simulink model "backup"  (R2017a)
settings: Solver=FixedStepDiscrete  StartTime=0.0  StopTime=inf  RelTol=1e-3  EnableMultiTasking=on
undefined symbols (not defined in the file or in its folder): fspecial, gray, Rec, SDTV, strel
libraries: simulink x11, visiontransforms x4, visionmorphops x3, visiontextngfix x3, visiongeotforms x2, visionsources x2, visionconversions x1, visionutilities x1, dspvision x1, visionstatistics x1, visionfilter x1
settings Model: FPTRunName=Active  Creator=The MathWorks, Inc.  LastModifiedBy=Pection
settings DataIOCC: LimitDataPoints=on  SaveFormat=StructureWithTime  SaveOutput=off  SignalLogging=off  SaveTime=off
settings OptimizationCC: ExpressionDepthLimit=2147483647  InitFltsAndDblsToZero=on  EfficientMapNaN2IntZero=off  LifeSpan=inf
settings DebuggingCC: UnderspecifiedInitializationDetection=Classic  MergeDetectMultiDrivingBlocksExec=none  SolverPrmCheckMsg=warning  ParameterPrecisionLossMsg=none  FcnCallInpInsideContextMsg=warning  StateNameClashWarn=warning  SFUnexpectedBacktrackingDiag=warning  SFNoUnconditionalDefaultTransitionDiag=warning  SFExecutionAtInitializationDiag=none
settings HardwareCC: ProdBitPerPointer=32  ProdBitPerSizeT=32  ProdBitPerPtrDiffT=32  ProdLargestAtomicFloat=None  ProdIntDivRoundTo=Undefined  ProdEndianess=Unspecified  ProdWordSize=32  ProdHWDeviceType=32-bit Generic  TargetBitPerPointer=64  TargetBitPerSizeT=64  TargetBitPerPtrDiffT=64  TargetLongLongMode=on  TargetIntDivRoundTo=Zero  TargetEndianess=LittleEndian  TargetWordSize=64  TargetHWDeviceType=Generic->MATLAB Host Computer  ProdEqTarget=off
settings ModelReferenceCC: PropagateSignalLabelsOutOfModel=off
settings SFSimCC: SimParseCustomCode=off
settings GRTTargetCC: TargetLangStandard=C89/C90 (ANSI)  GeneratePreprocessorConditionals=Disable all  CombineOutputUpdateFcns=off  GRTInterface=on
settings ConfigComp: CovMetricSettings=dw  CovHtmlReporting=on  CovSaveCumulativeToWorkspaceVar=on  CovSaveSingleToWorkspaceVar=on  CovExternalEMLEnable=off  CovSFcnEnable=off

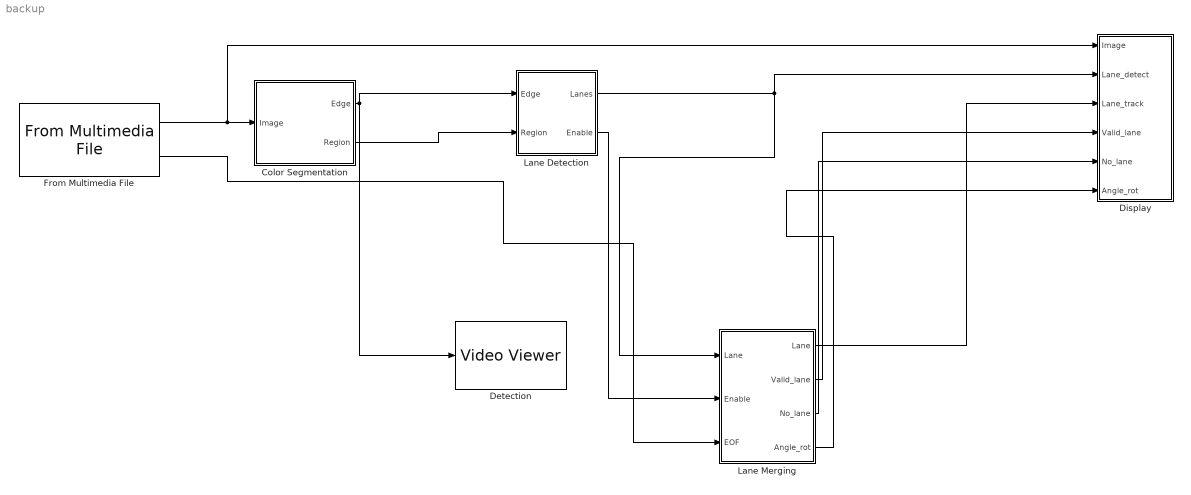
== system backup ==
  Color Segmentation : Subsystem
  Detection : VideoViewer  colormapValue=gray(256)  FigPos=[1 1038 1920 938]  trueSizedOnce=on
  Display : Subsystem
  From Multimedia File : dspvision/From Multimedia File  inputFilename=C:\Users\Pection\Desktop\vipunmarkedroad.avi  loop=on  numPlays=inf  outputStreams=Video only  videoDataType=single  audioDataType=int16  inheritSampleTime=off  userDefinedSampleTime=1/30  noAudioOutput=off  isIntensityVideo=off  fourcc=RGB  colorVideoFormat=One multidimensional signal  outputEOF=on  dataOrg=Column-major  audioFrameSize=1024  computeAudioFrameSize=off  outSamplingMode=Frame based
      settings: SourceProductBaseCode=VP
  Lane Detection : Subsystem
  Lane Merging : Subsystem
  wires:
  From Multimedia File/1 -> Display/1(Image), Color Segmentation/1(Image)
  Color Segmentation/2(Region) -> Lane Detection/2(Region)
  From Multimedia File/2 -> Lane Merging/3(EOF)
  Lane Detection/1(Lanes) -> Display/2(Lane_detect), Lane Merging/1(Lane)
  Lane Detection/2(Enable) -> Lane Merging/2(Enable)
  Lane Merging/1("Lane ") -> Display/3(Lane_track)
  Lane Merging/2(Valid_lane) -> Display/4(Valid_lane)
  Lane Merging/3(No_lane) -> Display/5(No_lane)
  Lane Merging/4(Angle_rot) -> Display/6(Angle_rot)
  Color Segmentation/1(Edge) -> Detection/1, Lane Detection/1(Edge)

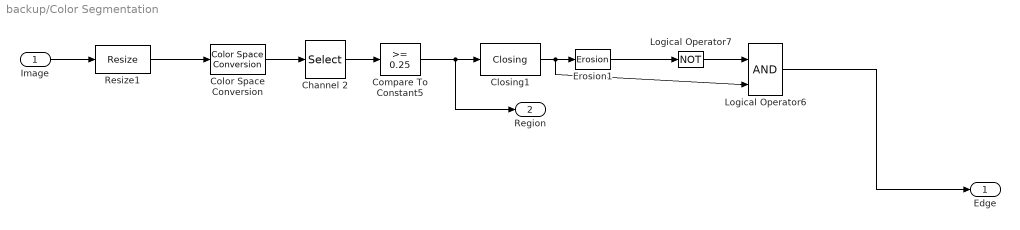
== system backup/Color Segmentation ==
  Image : Inport
  Channel 2 : Selector  NumberOfDimensions=3  InputPortWidth=3  IndexOptions=Select all,Select all,Index vector (dialog)  Indices=[1 3],1,[2]  OutputSizes=1,1,1
  Closing1 : visionmorphops/Closing  nhoodsrc=Specify via dialog  strel=strel('disk', 2)
      settings: SourceProductName=Computer Vision System Toolbox  SourceProductBaseCode=VP
  Color Space Conversion : visionconversions/Color Space  Conversion  conversion=Obsolete  conversionActive=R'G'B' to HSV  wp_str=D65  rec=Rec. 601 (SDTV)  sys=1125/60/2:1  imagePorts=One multidimensional signal
      settings: SourceProductName=Computer Vision System Toolbox
  Compare To Constant5 : simulink/Logic and Bit Operations/Compare To Constant  relop=>=  const=0.25  OutDataTypeStr=boolean  ZeroCross=off
  Erosion1 : visionmorphops/Erosion  nhoodsrc=Specify via dialog  strel=ones(3)
      settings: SourceProductName=Computer Vision System Toolbox  SourceProductBaseCode=VP
  Logical Operator6 : Logic  IconShape=distinctive  AllPortsSameDT=off  OutDataTypeStr=boolean
  Logical Operator7 : Logic  Operator=NOT  IconShape=distinctive  AllPortsSameDT=off  OutDataTypeStr=boolean
  Resize1 : visiongeotforms/Resize  specify=Output size as a percentage of input size  rfactor=50  outCols=25  outRows=25  outRowsCols=[120 160]  interp_method=Nearest neighbor  antialias=off  useROI=off  roiFlag=off  prodOutputMode=Binary point scaling  prodOutputWordLength=32  prodOutputFracLength=10  roundingMode=Nearest  overflowMode=on
      settings: AttributesFormatString=Downsample the\ninput image to\nreduce computation.  SourceProductName=Computer Vision System Toolbox  SourceProductBaseCode=VP
  Edge : Outport
  Region : Outport  Port=2
  wires:
  Color Space Conversion/1 -> Channel 2/1
  Channel 2/1 -> Compare To Constant5/1
  Closing1/1 -> Erosion1/1, Logical Operator6/2
  Logical Operator7/1 -> Logical Operator6/1
  Erosion1/1 -> Logical Operator7/1
  Compare To Constant5/1 -> Region/1, Closing1/1
  Image/1 -> Resize1/1
  Logical Operator6/1 -> Edge/1
  Resize1/1 -> Color Space Conversion/1

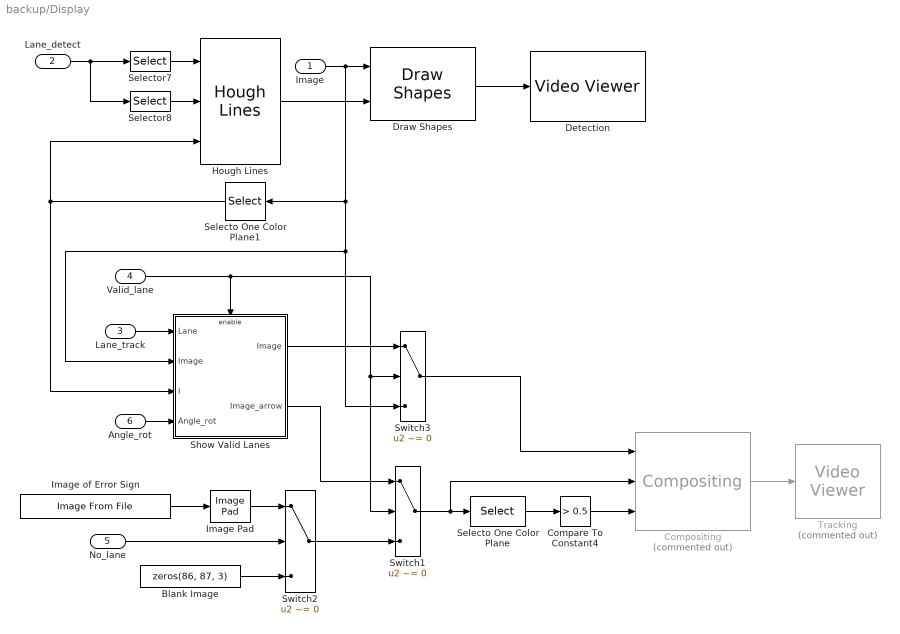
== system backup/Display ==
  Image : Inport
  Lane_detect : Inport  Port=2
  Lane_track : Inport  Port=3
  Valid_lane : Inport  Port=4
  No_lane : Inport  Port=5
  Angle_rot : Inport  Port=6
  Blank Image : Constant  Value=zeros(86, 87, 3)  OutDataTypeStr=Inherit: Inherit via back propagation
  Compare To Constant4 : simulink/Logic and Bit Operations/Compare To Constant  relop=>  const=0.5  OutDataTypeStr=uint8  ZeroCross=off
  Compositing : visiontextngfix/Compositing  Commented=on  operation=Binary mask  bFacSrc=Specify via dialog  mFacSrc=Input port  bFactor=0.75  mFactor=1  source=Specify via dialog  coordinates=[110 140]  prodOutputMode=Binary point scaling  prodOutputWordLength=32  prodOutputFracLength=10  roundingMode=Floor  overflowMode=off
      settings: SourceProductName=Computer Vision System Toolbox  SourceProductBaseCode=VP
  Detection : VideoViewer  colormapValue=gray(256)  FigPos=[169 782 575 518]  trueSizedOnce=on
  Draw Shapes : visiontextngfix/Draw Shapes  shape=Lines  fill=off  lineWidth=1  fillClrSource=Specify via dialog  display=User-specified value  intensity=200  color=[1 1 0; 1 0 1]  opacity=0.6  viewport=Entire image  antialiasing=off  inType=Obsolete  imagePorts=One multidimensional signal  prodOutputMode=Binary point scaling  prodOutputWordLength=32  prodOutputFracLength=14  memoryMode=Specify word length  memoryWordLength=16  memoryFracLength=15  roundingMode=Floor  overflowMode=off
      settings: SourceProductName=Computer Vision System Toolbox
  Hough Lines : visiontransforms/Hough Lines  sineCompMethod=Trigonometric function  thetaRes=pi/180  firstCoeffMode=Specify word length  firstCoeffWordLength=16  firstCoeffFracLength=15  prodOutputMode=Binary point scaling  prodOutputWordLength=32  prodOutputFracLength=16  roundingMode=Nearest  overflowMode=on
      settings: SourceProductName=Computer Vision System Toolbox  SourceProductBaseCode=VP
  Image Pad : visionutilities/Image Pad  method=Constant  valSrc=Specify via dialog  value=0  spec=Output size  rowDirection=Right  outRowsMode=User-specified  rowSize=86  outColSize=87  colDirection=Bottom  outColsMode=User-specified  colSize=87  outRowSize=86  trunc_flag=None
      settings: SourceProductName=Computer Vision System Toolbox  SourceProductBaseCode=VP
  Image of Error Sign : visionsources/Image From File  Tag=vipblks_nd  FileName=viperrorsign.png  imagePorts=One multidimensional signal  Ts=inf  ImageDataType=single  Signed=on  WordLength=16  sdImageDataType=uint(8)  FractionLengthMode=User-defined  FractionLength=15  OutPortLabels=R|G|B
      settings: SourceProductName=Computer Vision System Toolbox
  Selecto One Color Plane : Selector  NumberOfDimensions=3  IndexMode=Zero-based  InputPortWidth=3  IndexOptions=Select all,Select all,Index vector (dialog)  Indices=[1 3],1,0  OutputSizes=1,1,1
  Selecto One Color Plane1 : Selector  NumberOfDimensions=3  IndexMode=Zero-based  InputPortWidth=3  IndexOptions=Select all,Select all,Index vector (dialog)  Indices=[1 3],1,0  OutputSizes=1,1,1
  Selector7 : Selector  NumberOfDimensions=2  IndexMode=Zero-based  InputPortWidth=2  IndexOptions=Index vector (dialog),Select all  Indices=1,0  OutputSizes=1,1
  Selector8 : Selector  NumberOfDimensions=2  IndexMode=Zero-based  InputPortWidth=2  IndexOptions=Index vector (dialog),Select all  Indices=0,0  OutputSizes=1,1
  Show Valid Lanes : Subsystem
  Switch1 : Switch  Criteria=u2 ~= 0
  Switch2 : Switch  Criteria=u2 ~= 0
  Switch3 : Switch  Criteria=u2 ~= 0
  Tracking : VideoViewer  Commented=on  colormapValue=gray(256)  FigPos=[852 826 725 493]  trueSizedOnce=on
  wires:
  Hough Lines/1 -> Draw Shapes/2
  Image/1 -> Draw Shapes/1, Switch3/3, Show Valid Lanes/2(Image), Selecto One Color Plane1/1
  Draw Shapes/1 -> Detection/1
  Selector7/1 -> Hough Lines/1
  Selector8/1 -> Hough Lines/2
  Selecto One Color Plane/1 -> Compare To Constant4/1
  Compare To Constant4/1 -> Compositing/3
  Blank Image/1 -> Switch2/3
  Image of Error Sign/1 -> Image Pad/1
  Switch2/1 -> Switch1/3
  Compositing/1 -> Tracking/1
  Image Pad/1 -> Switch2/1
  Lane_detect/1 -> Selector7/1, Selector8/1
  Switch3/1 -> Compositing/1
  Show Valid Lanes/1("Image ") -> Switch3/1
  Show Valid Lanes/2(Image_arrow) -> Switch1/1
  No_lane/1 -> Switch2/2
  Switch1/1 -> Selecto One Color Plane/1, Compositing/2
  Lane_track/1 -> Show Valid Lanes/1(Lane)
  Angle_rot/1 -> Show Valid Lanes/4(Angle_rot)
  Valid_lane/1 -> Show Valid Lanes/Enable, Switch3/2, Switch1/2
  Selecto One Color Plane1/1 -> Hough Lines/3, Show Valid Lanes/3(I)

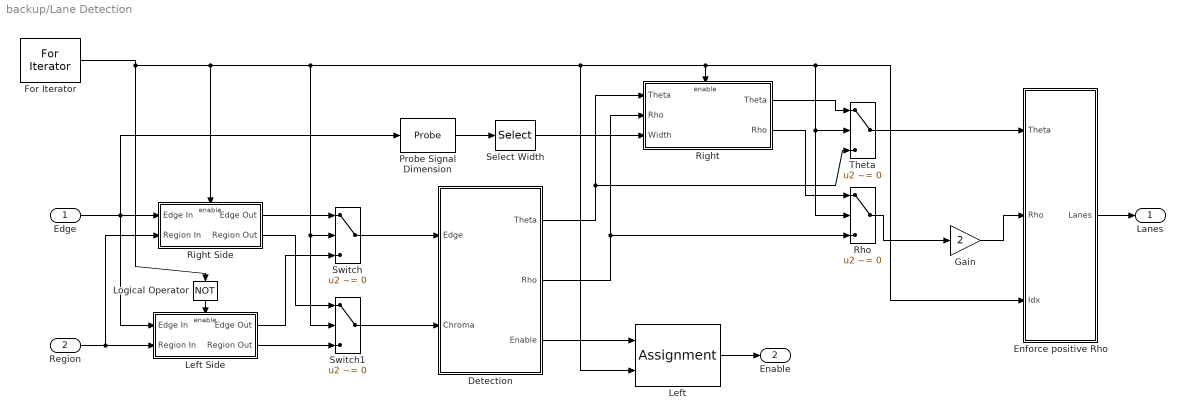
== system backup/Lane Detection ==
  Edge : Inport
  Region : Inport  Port=2
  Detection : Subsystem
  Enforce positive Rho : Subsystem
  For Iterator : ForIterator  IterationLimit=2  IndexMode=Zero-based  IterationVariableDataType=int8
  Gain : Gain  Gain=2
  Left : Assignment  NumberOfDimensions=2  IndexMode=Zero-based  OutputInitialize=Specify size for each dimension in table  IndexOptions=Assign all,Index vector (port)  Indices=1,1  OutputSizes=1,2
  Left Side : Subsystem  TreatAsAtomicUnit=on
  Logical Operator : Logic  Operator=NOT  IconShape=distinctive  AllPortsSameDT=off  OutDataTypeStr=boolean
  Probe Signal Dimension : Probe  ProbeWidth=off  ProbeSampleTime=off  ProbeComplexSignal=off  ProbeSignalDimensions=on  ProbeDimensionsDataType=single
  Rho : Switch  Criteria=u2 ~= 0
  Right : Subsystem  TreatAsAtomicUnit=on
  Right Side : Subsystem  TreatAsAtomicUnit=on
  Select Width : Selector  IndexMode=Zero-based  InputPortWidth=2  IndexOptions=Index vector (dialog)  Indices=1  OutputSizes=1
  Switch : Switch  Criteria=u2 ~= 0
  Switch1 : Switch  Criteria=u2 ~= 0
  Theta : Switch  Criteria=u2 ~= 0
  Lanes : Outport
  Enable : Outport  Port=2
  wires:
  Logical Operator/1 -> Left Side/Enable
  For Iterator/1 -> Logical Operator/1, Right Side/Enable, Switch/2, Switch1/2, Right/Enable, Enforce positive Rho/3(Idx), Theta/2, Rho/2, Left/2
  Edge/1 -> Right Side/1(Edge In), Left Side/1(Edge In), Probe Signal Dimension/1
  Region/1 -> Left Side/2(Region In), Right Side/2(Region In)
  Switch/1 -> Detection/1(Edge)
  Right Side/1(Edge Out) -> Switch/1
  Left Side/1(Edge Out) -> Switch/3
  Switch1/1 -> Detection/2(Chroma)
  Right Side/2(Region Out) -> Switch1/1
  Left Side/2("Region Out ") -> Switch1/3
  Left/1 -> Enable/1
  Right/1("Theta ") -> Theta/1
  Right/2("Rho ") -> Rho/1
  Enforce positive Rho/1(Lanes) -> Lanes/1
  Detection/3(Enable) -> Left/1
  Theta/1 -> Enforce positive Rho/1(Theta)
  Rho/1 -> Gain/1
  Detection/1(Theta) -> Right/1(Theta), Theta/3
  Detection/2(Rho) -> Right/2(Rho), Rho/3
  Gain/1 -> Enforce positive Rho/2(Rho)
  Probe Signal Dimension/1 -> Select Width/1
  Select Width/1 -> Right/3(Width)

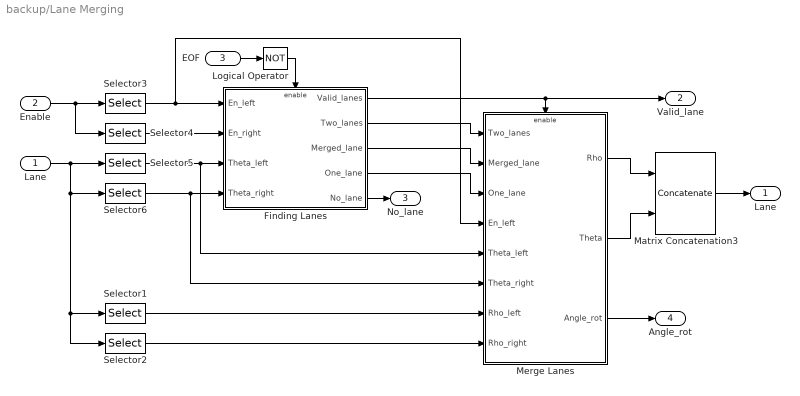
== system backup/Lane Merging ==
  Lane : Inport
  Enable : Inport  Port=2
  EOF : Inport  Port=3
  Finding Lanes : Subsystem  mask{appearTime=4}
      mask prompts: appearTime "Minimum number of frames a lane must be detected to become a valid lane:"
  Logical Operator : Logic  Operator=NOT  IconShape=distinctive  AllPortsSameDT=off  OutDataTypeStr=boolean
  Matrix Concatenation3 : Concatenate  Mode=Multidimensional array
  Merge Lanes : Subsystem
  Selector1 : Selector  NumberOfDimensions=2  IndexMode=Zero-based  InputPortWidth=2  IndexOptions=Index vector (dialog),Index vector (dialog)  Indices=0,0  OutputSizes=1,1
  Selector2 : Selector  NumberOfDimensions=2  IndexMode=Zero-based  InputPortWidth=2  IndexOptions=Index vector (dialog),Index vector (dialog)  Indices=0,1  OutputSizes=1,1
  Selector3 : Selector  IndexMode=Zero-based  InputPortWidth=2  IndexOptions=Index vector (dialog)  Indices=0  OutputSizes=1
  Selector4 : Selector  IndexMode=Zero-based  InputPortWidth=2  IndexOptions=Index vector (dialog)  Indices=1  OutputSizes=1
  Selector5 : Selector  NumberOfDimensions=2  IndexMode=Zero-based  InputPortWidth=2  IndexOptions=Index vector (dialog),Index vector (dialog)  Indices=1,0  OutputSizes=1,1
  Selector6 : Selector  NumberOfDimensions=2  IndexMode=Zero-based  InputPortWidth=2  IndexOptions=Index vector (dialog),Index vector (dialog)  Indices=1,1  OutputSizes=1,1
  "Lane " : Outport
  Valid_lane : Outport  Port=2
  No_lane : Outport  Port=3
  Angle_rot : Outport  Port=4
  wires:
  Enable/1 -> Selector3/1, Selector4/1
  Finding Lanes/2(Two_lanes) -> Merge Lanes/1(Two_lanes)
  Finding Lanes/3(Merged_lane) -> Merge Lanes/2(Merged_lane)
  Finding Lanes/4(One_lane) -> Merge Lanes/3(One_lane)
  EOF/1 -> Logical Operator/1
  Logical Operator/1 -> Finding Lanes/Enable
  Selector3/1 -> Finding Lanes/1(En_left), Merge Lanes/4(En_left)
  Selector4/1 -> Finding Lanes/2(En_right)
  Lane/1 -> Selector5/1, Selector6/1, Selector2/1, Selector1/1
  Selector5/1 -> Finding Lanes/3(Theta_left), Merge Lanes/5(Theta_left)
  Selector6/1 -> Finding Lanes/4(Theta_right), Merge Lanes/6(Theta_right)
  Finding Lanes/5(No_lane) -> No_lane/1
  Merge Lanes/3(Angle_rot) -> Angle_rot/1
  Finding Lanes/1(Valid_lanes) -> Merge Lanes/Enable, Valid_lane/1
  Merge Lanes/1("Rho ") -> Matrix Concatenation3/1
  Merge Lanes/2("Theta ") -> Matrix Concatenation3/2
  Matrix Concatenation3/1 -> "Lane "/1
  Selector1/1 -> Merge Lanes/7(Rho_left)
  Selector2/1 -> Merge Lanes/8(Rho_right)

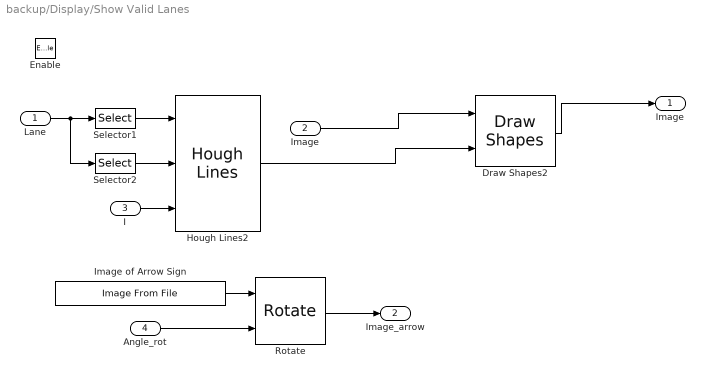
== system backup/Display/Show Valid Lanes ==
  Lane : Inport
  Image : Inport  Port=2
  I : Inport  Port=3
  Angle_rot : Inport  Port=4
  Enable : EnablePort  StatesWhenEnabling=reset  PropagateVarSize=During execution
  Draw Shapes2 : visiontextngfix/Draw Shapes  shape=Lines  fill=off  lineWidth=1  fillClrSource=Specify via dialog  display=User-specified value  intensity=200  color=[1 1 0; 1 0 1; 0 1 1]  opacity=0.6  viewport=Entire image  antialiasing=off  inType=Obsolete  imagePorts=One multidimensional signal  prodOutputMode=Binary point scaling  prodOutputWordLength=32  prodOutputFracLength=14  memoryMode=Specify word length  memoryWordLength=16  memoryFracLength=15  roundingMode=Floor  overflowMode=off
      settings: SourceProductName=Computer Vision System Toolbox
  Hough Lines2 : visiontransforms/Hough Lines  sineCompMethod=Trigonometric function  thetaRes=pi/180  firstCoeffMode=Specify word length  firstCoeffWordLength=16  firstCoeffFracLength=15  prodOutputMode=Binary point scaling  prodOutputWordLength=32  prodOutputFracLength=16  roundingMode=Nearest  overflowMode=on
      settings: SourceProductName=Computer Vision System Toolbox  SourceProductBaseCode=VP
  Image of Arrow Sign : visionsources/Image From File  Tag=vipblks_nd  FileName=viparrowsign.png  imagePorts=One multidimensional signal  Ts=inf  ImageDataType=single  Signed=on  WordLength=16  sdImageDataType=uint(8)  FractionLengthMode=User-defined  FractionLength=15  OutPortLabels=R|G|B
      settings: SourceProductName=Computer Vision System Toolbox
  Rotate : visiongeotforms/Rotate  outSizeR=Expanded to fit rotated input image  src_angle=Input port  unit_angle=Degrees  angle=pi/6  maxAngle=pi  dispImage=Center  method=Trigonometric function  fillVal=0  interpMethod=Bilinear  prodOutputMode=Binary point scaling  prodOutputWordLength=32  prodOutputFracLength=10  roundingMode=Nearest  overflowMode=on
      settings: SourceProductName=Computer Vision System Toolbox
  Selector1 : Selector  NumberOfDimensions=2  IndexMode=Zero-based  InputPortWidth=2  IndexOptions=Index vector (dialog),Select all  Indices=1,0  OutputSizes=1,1
  Selector2 : Selector  NumberOfDimensions=2  IndexMode=Zero-based  InputPortWidth=2  IndexOptions=Index vector (dialog),Select all  Indices=0,0  OutputSizes=1,1
  "Image " : Outport
  Image_arrow : Outport  Port=2
  wires:
  Hough Lines2/1 -> Draw Shapes2/2
  Image of Arrow Sign/1 -> Rotate/1
  Lane/1 -> Selector1/1, Selector2/1
  Selector1/1 -> Hough Lines2/1
  Selector2/1 -> Hough Lines2/2
  Angle_rot/1 -> Rotate/2
  Image/1 -> Draw Shapes2/1
  I/1 -> Hough Lines2/3
  Draw Shapes2/1 -> "Image "/1
  Rotate/1 -> Image_arrow/1

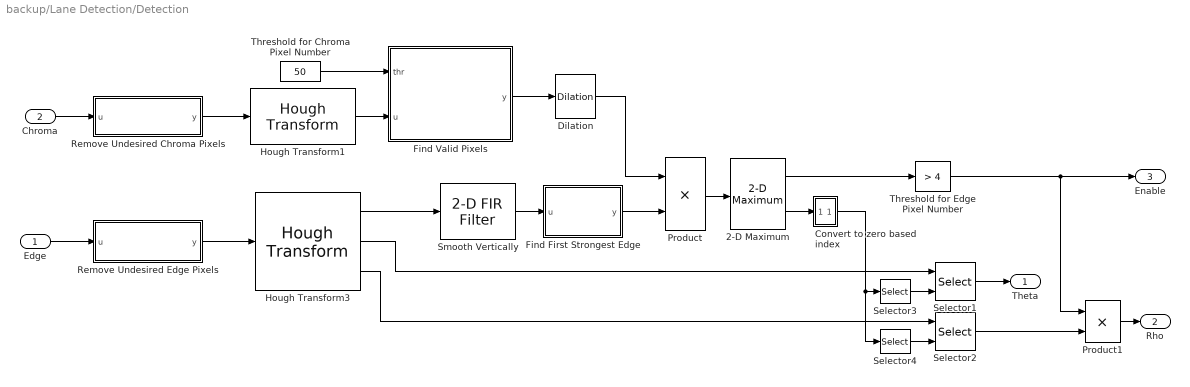
== system backup/Lane Detection/Detection ==
  Edge : Inport
  Chroma : Inport  Port=2
  2-D Maximum : visionstatistics/2-D Maximum  fcn=Value and Index  reset=None  indexBase=One  operateOver=Entire input  Dimension=1  colComp=on  operation=maximum  roiEnable=off  roiType=Rectangles  roiPortion=Entire ROI  roiOutput=Individual statistics for each ROI  roiFlag=off  accumDataTypeStr=Inherit: Same as product output  accumLastDataTypeStr=Inherit: Same as product output  roundingMode=Floor  overflowMode=off
      settings: SourceProductName=Computer Vision System Toolbox  SourceProductBaseCode=VP
  "Convert to zero based index " : Subsystem
  Dilation : visionmorphops/Dilation  nhoodsrc=Specify via dialog  strel=ones(3, 1)
      settings: SourceProductName=Computer Vision System Toolbox  SourceProductBaseCode=VP
  Find First Strongest Edge : MATLAB Function  TreatAsAtomicUnit=on
  Find Valid Pixels : MATLAB Function  TreatAsAtomicUnit=on
      settings: AttributesFormatString=Find valid pixels in each of the angles.
  Hough Transform1 : visiontransforms/Hough Transform  theta_res=pi/90  rho_res=2  out_theta_rho=off  outdtmode=single  firstCoeffMode=Binary point scaling  firstCoeffWordLength=16  firstCoeffFracLength=14  secondCoeffMode=Binary point scaling  secondCoeffWordLength=32  secondCoeffFracLength=16  outputMode=Binary point scaling  outputWordLength=16  outputFracLength=0  accumMode=Binary point scaling  accumWordLength=32  accumFracLength=20  prodOutputMode=Binary point scaling  prodOutputWordLength=32  prodOutputFracLength=20  memoryMode=Binary point scaling  memoryWordLength=32  memoryFracLength=16  roundingMode=Nearest  overflowMode=on
      settings: SourceProductName=Computer Vision System Toolbox  SourceProductBaseCode=VP
  Hough Transform3 : visiontransforms/Hough Transform  theta_res=pi/90  rho_res=2  out_theta_rho=on  outdtmode=single  firstCoeffMode=Binary point scaling  firstCoeffWordLength=16  firstCoeffFracLength=14  secondCoeffMode=Binary point scaling  secondCoeffWordLength=32  secondCoeffFracLength=16  outputMode=Binary point scaling  outputWordLength=16  outputFracLength=0  accumMode=Binary point scaling  accumWordLength=32  accumFracLength=20  prodOutputMode=Binary point scaling  prodOutputWordLength=32  prodOutputFracLength=20  memoryMode=Binary point scaling  memoryWordLength=32  memoryFracLength=16  roundingMode=Nearest  overflowMode=on
      settings: SourceProductName=Computer Vision System Toolbox  SourceProductBaseCode=VP
  Product : Product  RndMeth=Zero
  Product1 : Product  RndMeth=Zero
  Remove Undesired Chroma Pixels : MATLAB Function  TreatAsAtomicUnit=on
  Remove Undesired Edge Pixels : MATLAB Function  TreatAsAtomicUnit=on
  Selector1 : Selector  IndexMode=Zero-based  IndexOptions=Index vector (port)  Indices=[1 3]  OutputSizes=1
  Selector2 : Selector  IndexMode=Zero-based  IndexOptions=Index vector (port)  Indices=[1 3]  OutputSizes=1
  Selector3 : Selector  IndexMode=Zero-based  InputPortWidth=2  IndexOptions=Index vector (dialog)  Indices=1  OutputSizes=1
  Selector4 : Selector  IndexMode=Zero-based  InputPortWidth=2  IndexOptions=Index vector (dialog)  Indices=0  OutputSizes=1
  Smooth Vertically : visionfilter/2-D FIR Filter  separable=off  filtSrc=Specify via dialog  filterMtrx=fspecial('gaussian', [5, 1], 1.5)  verticalFilter=fspecial('gaussian', [7, 1] ,2)  horizontalFilter=1  outSize=Same as input port I  padType=Replicate  padSrc=Specify via dialog  padVal=0  method=Convolution  firstCoeffMode=Specify word length  firstCoeffWordLength=16  firstCoeffFracLength=17  firstCoeffSignedness=Signed  firstCoeffDataTypeStr=fixdt(1,16)  firstCoeffLastDataTypeStr=fixdt(1,16)  firstCoeffMin=[]  firstCoeffMax=[]  outputSignedness=Auto  outputMin=[]  outputMax=[]  accumDataTypeStr=Inherit: Same as product output  accumLastDataTypeStr=Inherit: Same as product output  prodOutputMode=Binary point scaling  prodOutputWordLength=32  prodOutputFracLength=10  prodOutputDataTypeStr=fixdt([],32,10)  prodOutputLastDataTypeStr=fixdt([],32,10)  roundingMode=Floor  overflowMode=off
      settings: SourceProductName=Computer Vision System Toolbox  SourceProductBaseCode=VP
  Threshold for Chroma Pixel Number : Constant  Value=50
  Threshold for Edge Pixel Number : simulink/Logic and Bit Operations/Compare To Constant  relop=>  const=4  OutDataTypeStr=uint8  ZeroCross=off
  Theta : Outport
  Rho : Outport  Port=2
  Enable : Outport  Port=3
  wires:
  Remove Undesired Edge Pixels/1(y) -> Hough Transform3/1
  Hough Transform3/1 -> Smooth Vertically/1
  Hough Transform3/2 -> Selector1/1
  Hough Transform3/3 -> Selector2/1
  Selector3/1 -> Selector1/2
  Selector4/1 -> Selector2/2
  Smooth Vertically/1 -> Find First Strongest Edge/1(u)
  2-D Maximum/1 -> Threshold for Edge Pixel Number/1
  Selector1/1 -> Theta/1
  Edge/1 -> Remove Undesired Edge Pixels/1(u)
  Chroma/1 -> Remove Undesired Chroma Pixels/1(u)
  Threshold for Edge Pixel Number/1 -> Product1/1, Enable/1
  Product1/1 -> Rho/1
  Selector2/1 -> Product1/2
  Find First Strongest Edge/1(y) -> Product/2
  Product/1 -> 2-D Maximum/1
  Hough Transform1/1 -> Find Valid Pixels/2(u)
  Find Valid Pixels/1(y) -> Dilation/1
  Remove Undesired Chroma Pixels/1(y) -> Hough Transform1/1
  Threshold for Chroma Pixel Number/1 -> Find Valid Pixels/1(thr)
  Dilation/1 -> Product/1
  2-D Maximum/2 -> "Convert to zero based index "/1(In1)
  "Convert to zero based index "/1(Out1) -> Selector3/1, Selector4/1

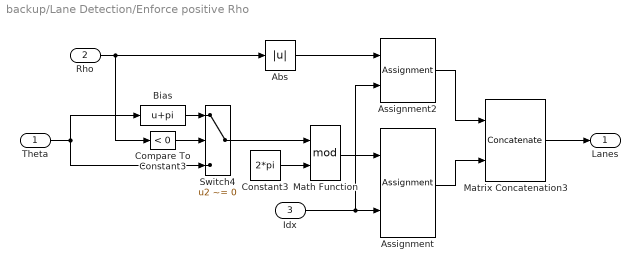
== system backup/Lane Detection/Enforce positive Rho ==
  Theta : Inport
  Rho : Inport  Port=2
  Idx : Inport  Port=3
  Abs : Abs
  Assignment : Assignment  NumberOfDimensions=2  IndexMode=Zero-based  OutputInitialize=Specify size for each dimension in table  IndexOptions=Assign all,Index vector (port)  Indices=1,1  OutputSizes=1,2
  Assignment2 : Assignment  NumberOfDimensions=2  IndexMode=Zero-based  OutputInitialize=Specify size for each dimension in table  IndexOptions=Assign all,Index vector (port)  Indices=1,1  OutputSizes=1,2
  Bias : Bias  Bias=pi
  Compare To Constant3 : simulink/Logic and Bit Operations/Compare To Constant  relop=<  const=0  OutDataTypeStr=uint8  ZeroCross=off
  Constant3 : Constant  Value=2*pi  OutDataTypeStr=Inherit: Inherit via back propagation
  Math Function : Math  Operator=mod  SaturateOnIntegerOverflow=on
  Matrix Concatenation3 : Concatenate  Mode=Multidimensional array
  Switch4 : Switch  Criteria=u2 ~= 0
  Lanes : Outport
  wires:
  Theta/1 -> Switch4/3, Bias/1
  Bias/1 -> Switch4/1
  Idx/1 -> Assignment/2, Assignment2/2
  Assignment/1 -> Matrix Concatenation3/2
  Assignment2/1 -> Matrix Concatenation3/1
  Math Function/1 -> Assignment/1
  Constant3/1 -> Math Function/2
  Switch4/1 -> Math Function/1
  Matrix Concatenation3/1 -> Lanes/1
  Compare To Constant3/1 -> Switch4/2
  Abs/1 -> Assignment2/1
  Rho/1 -> Abs/1, Compare To Constant3/1

== system backup/Lane Detection/Left Side ==
  Edge In : Inport
  Region In : Inport  Port=2
  Enable : EnablePort  PropagateVarSize=During execution
  Cut Left Edge : MATLAB Function  TreatAsAtomicUnit=on
      settings: AttributesFormatString=Cut the left part of the image.
  Cut Left Region : MATLAB Function  TreatAsAtomicUnit=on
      settings: AttributesFormatString=Cut the left part of the image.
  Edge Out : Outport
  "Region Out " : Outport  Port=2
  wires:
  Edge In/1 -> Cut Left Edge/1(u)
  Cut Left Edge/1(y) -> Edge Out/1
  Region In/1 -> Cut Left Region/1(u)
  Cut Left Region/1(y) -> "Region Out "/1

== system backup/Lane Detection/Right ==
  Theta : Inport
  Rho : Inport  Port=2
  Width : Inport  Port=3
  Enable : EnablePort  PropagateVarSize=During execution
  Add6 : Sum  Inputs=+-
  Add7 : Sum  Inputs=-+
  Constant10 : Constant  Value=pi  OutDataTypeStr=single
  Product1 : Product  RndMeth=Zero
  Trigonometric Function1 : Trigonometry  Operator=cos
  "Theta " : Outport
  "Rho " : Outport  Port=2
  wires:
  Trigonometric Function1/1 -> Product1/1
  Width/1 -> Product1/2
  Add6/1 -> "Theta "/1
  Theta/1 -> Trigonometric Function1/1, Add6/2
  Add7/1 -> "Rho "/1
  Product1/1 -> Add7/1
  Rho/1 -> Add7/2
  Constant10/1 -> Add6/1

== system backup/Lane Detection/Right Side ==
  Edge In : Inport
  Region In : Inport  Port=2
  Enable : EnablePort  PropagateVarSize=During execution
  Flip Right Edge : MATLAB Function  TreatAsAtomicUnit=on
      settings: AttributesFormatString=Cut and flip the right\npart of the image
  Flip Right Region : MATLAB Function  TreatAsAtomicUnit=on
      settings: AttributesFormatString=Cut and flip the right\npart of the image
  Edge Out : Outport
  Region Out : Outport  Port=2
  wires:
  Flip Right Edge/1(y) -> Edge Out/1
  Edge In/1 -> Flip Right Edge/1(u)
  Region In/1 -> Flip Right Region/1(u)
  Flip Right Region/1(y) -> Region Out/1

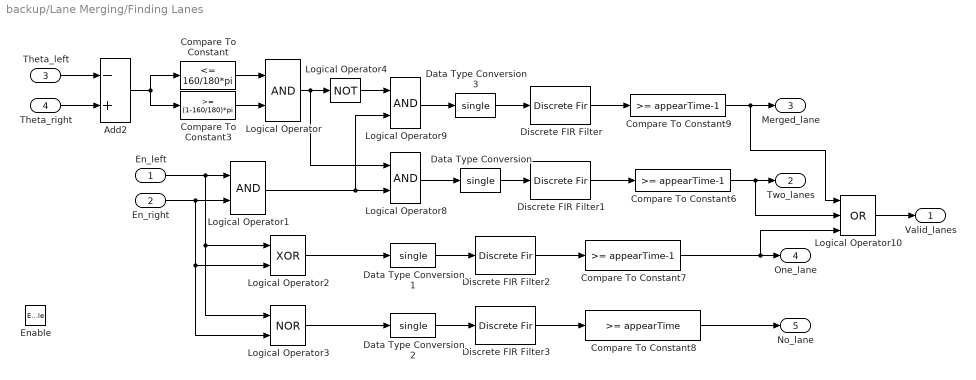
== system backup/Lane Merging/Finding Lanes ==
  En_left : Inport
  En_right : Inport  Port=2
  Theta_left : Inport  Port=3
  Theta_right : Inport  Port=4
  Enable : EnablePort  StatesWhenEnabling=reset  PropagateVarSize=During execution
  Add2 : Sum  Inputs=-+
  Compare To Constant : simulink/Logic and Bit Operations/Compare To Constant  relop=<=  const=160/180*pi  OutDataTypeStr=uint8  ZeroCross=off
  Compare To Constant3 : simulink/Logic and Bit Operations/Compare To Constant  relop=>=  const=(1-160/180)*pi  OutDataTypeStr=uint8  ZeroCross=off
  Compare To Constant6 : simulink/Logic and Bit Operations/Compare To Constant  relop=>=  const=appearTime-1  OutDataTypeStr=uint8  ZeroCross=off
  Compare To Constant7 : simulink/Logic and Bit Operations/Compare To Constant  relop=>=  const=appearTime-1  OutDataTypeStr=uint8  ZeroCross=off
  Compare To Constant8 : simulink/Logic and Bit Operations/Compare To Constant  relop=>=  const=appearTime  OutDataTypeStr=uint8  ZeroCross=off
  Compare To Constant9 : simulink/Logic and Bit Operations/Compare To Constant  relop=>=  const=appearTime-1  OutDataTypeStr=uint8  ZeroCross=off
  Data Type Conversion{,1..3} (4 alike) : DataTypeConversion  OutDataTypeStr=single
  Discrete FIR Filter : DiscreteFir  Coefficients=ones(1, appearTime)
  Discrete FIR Filter1 : DiscreteFir  Coefficients=ones(1, appearTime)
  Discrete FIR Filter2 : DiscreteFir  Coefficients=ones(1, appearTime)
  Discrete FIR Filter3 : DiscreteFir  Coefficients=ones(1, appearTime+1)
  Logical Operator{,1,8..9} (4 alike) : Logic  AllPortsSameDT=off  OutDataTypeStr=boolean
  Logical Operator10 : Logic  Operator=OR  Inputs=3  AllPortsSameDT=off  OutDataTypeStr=boolean
  Logical Operator2 : Logic  Operator=XOR  AllPortsSameDT=off  OutDataTypeStr=boolean
  Logical Operator3 : Logic  Operator=NOR  AllPortsSameDT=off  OutDataTypeStr=boolean
  Logical Operator4 : Logic  Operator=NOT  AllPortsSameDT=off  OutDataTypeStr=boolean
  Valid_lanes : Outport
  Two_lanes : Outport  Port=2
  Merged_lane : Outport  Port=3
  One_lane : Outport  Port=4
  No_lane : Outport  Port=5
  wires:
  Compare To Constant/1 -> Logical Operator/1
  Compare To Constant3/1 -> Logical Operator/2
  Discrete FIR Filter1/1 -> Compare To Constant6/1
  Discrete FIR Filter2/1 -> Compare To Constant7/1
  Logical Operator1/1 -> Logical Operator8/2, Logical Operator9/2
  Logical Operator8/1 -> Data Type Conversion/1
  Logical Operator4/1 -> Logical Operator9/1
  Discrete FIR Filter3/1 -> Compare To Constant8/1
  Logical Operator3/1 -> Data Type Conversion2/1
  Compare To Constant6/1 -> Two_lanes/1, Logical Operator10/2
  Compare To Constant7/1 -> One_lane/1, Logical Operator10/3
  Data Type Conversion/1 -> Discrete FIR Filter1/1
  Data Type Conversion1/1 -> Discrete FIR Filter2/1
  Data Type Conversion2/1 -> Discrete FIR Filter3/1
  Discrete FIR Filter/1 -> Compare To Constant9/1
  Data Type Conversion3/1 -> Discrete FIR Filter/1
  Logical Operator9/1 -> Data Type Conversion3/1
  Compare To Constant9/1 -> Merged_lane/1, Logical Operator10/1
  Logical Operator2/1 -> Data Type Conversion1/1
  Theta_left/1 -> Add2/1
  Theta_right/1 -> Add2/2
  En_left/1 -> Logical Operator1/1, Logical Operator2/1, Logical Operator3/1
  En_right/1 -> Logical Operator1/2, Logical Operator2/2, Logical Operator3/2
  Logical Operator10/1 -> Valid_lanes/1
  Compare To Constant8/1 -> No_lane/1
  Logical Operator/1 -> Logical Operator4/1, Logical Operator8/1
  Add2/1 -> Compare To Constant/1, Compare To Constant3/1

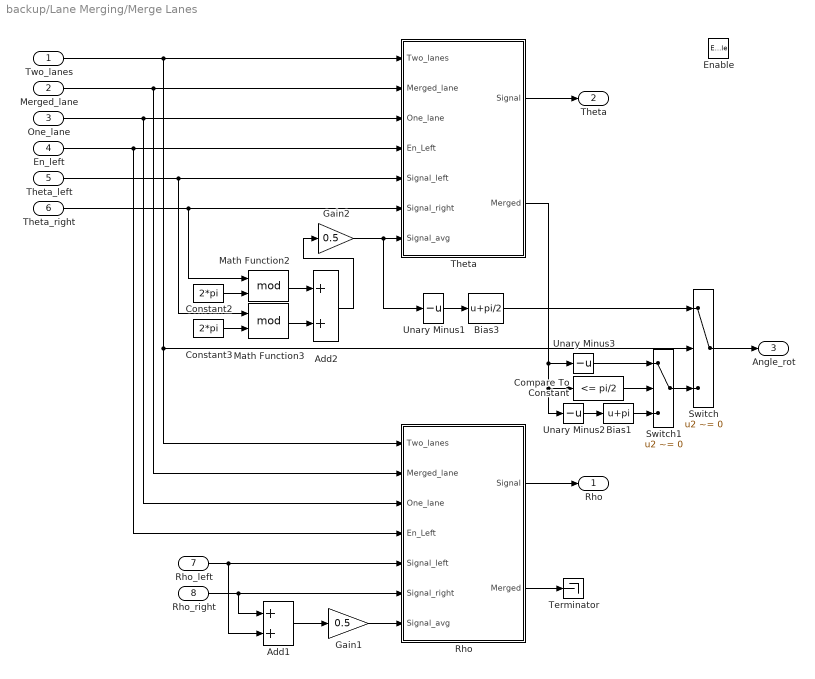
== system backup/Lane Merging/Merge Lanes ==
  Two_lanes : Inport
  Merged_lane : Inport  Port=2
  One_lane : Inport  Port=3
  En_left : Inport  Port=4
  Theta_left : Inport  Port=5
  Theta_right : Inport  Port=6
  Rho_left : Inport  Port=7
  Rho_right : Inport  Port=8
  Enable : EnablePort  PropagateVarSize=During execution
  Add1 : Sum
  Add2 : Sum
  Bias1 : Bias  Bias=pi
  Bias3 : Bias  Bias=pi/2
  Compare To Constant : simulink/Logic and Bit Operations/Compare To Constant  relop=<=  const=pi/2  OutDataTypeStr=uint8  ZeroCross=off
  Constant2 : Constant  Value=2*pi  OutDataTypeStr=Inherit: Inherit via back propagation
  Constant3 : Constant  Value=2*pi  OutDataTypeStr=Inherit: Inherit via back propagation
  Gain1 : Gain  Gain=0.5
  Gain2 : Gain  Gain=0.5
  Math Function2 : Math  Operator=mod  SaturateOnIntegerOverflow=on
  Math Function3 : Math  Operator=mod  SaturateOnIntegerOverflow=on
  Rho : Subsystem
  Switch : Switch  Criteria=u2 ~= 0
  Switch1 : Switch  Criteria=u2 ~= 0
  Terminator : Terminator
  Theta : Subsystem
  Unary Minus1 : UnaryMinus
  Unary Minus2 : UnaryMinus
  Unary Minus3 : UnaryMinus
  "Rho " : Outport
  "Theta " : Outport  Port=2
  Angle_rot : Outport  Port=3
  wires:
  Theta/2("Merged ") -> Compare To Constant/1, Unary Minus2/1, Unary Minus3/1
  Two_lanes/1 -> Theta/1(Two_lanes), Rho/1(Two_lanes), Switch/2
  Merged_lane/1 -> Theta/2(Merged_lane), Rho/2(Merged_lane)
  One_lane/1 -> Theta/3(One_lane), Rho/3(One_lane)
  En_left/1 -> Theta/4(En_Left), Rho/4(En_Left)
  Theta_left/1 -> Theta/5(Signal_left), Math Function3/1
  Theta_right/1 -> Theta/6(Signal_right), Math Function2/1
  Rho_left/1 -> Rho/5(Signal_left), Add1/2
  Rho_right/1 -> Rho/6(Signal_right), Add1/1
  Add1/1 -> Gain1/1
  Gain1/1 -> Rho/7(Signal_avg)
  Rho/2("Merged ") -> Terminator/1
  Theta/1(Signal) -> "Theta "/1
  Rho/1(Signal) -> "Rho "/1
  Gain2/1 -> Theta/7(Signal_avg), Unary Minus1/1
  Constant2/1 -> Math Function2/2
  Constant3/1 -> Math Function3/2
  Math Function2/1 -> Add2/1
  Math Function3/1 -> Add2/2
  Add2/1 -> Gain2/1
  Switch1/1 -> Switch/3
  Compare To Constant/1 -> Switch1/2
  Bias1/1 -> Switch1/3
  Bias3/1 -> Switch/1
  Unary Minus1/1 -> Bias3/1
  Unary Minus2/1 -> Bias1/1
  Unary Minus3/1 -> Switch1/1
  Switch/1 -> Angle_rot/1

== system backup/Lane Detection/Detection/Convert to zero based index  ==
  In1 : Inport
  Constant : Constant
  Selector : Selector  NumberOfDimensions=2  InputPortWidth=3  IndexOptions=Select all,Index vector (dialog)  Indices=[1 3],[2 1]  OutputSizes=1,1
  Subtract : Sum  Inputs=+-
  Out1 : Outport
  wires:
  Selector/1 -> Subtract/1
  Constant/1 -> Subtract/2
  In1/1 -> Selector/1
  Subtract/1 -> Out1/1

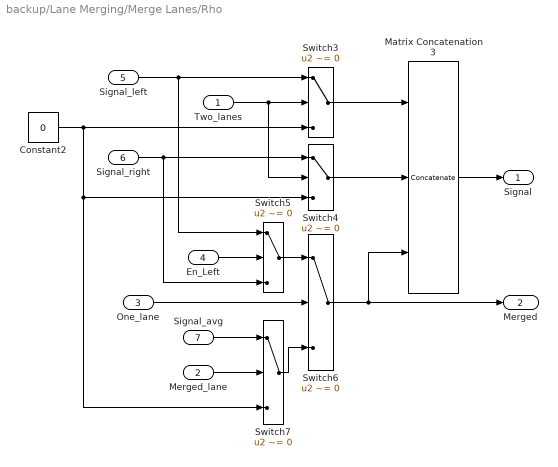
== system backup/Lane Merging/Merge Lanes/Rho ==
  Two_lanes : Inport
  Merged_lane : Inport  Port=2
  One_lane : Inport  Port=3
  En_Left : Inport  Port=4
  Signal_left : Inport  Port=5
  Signal_right : Inport  Port=6
  Signal_avg : Inport  Port=7
  Constant2 : Constant  Value=0  OutDataTypeStr=Inherit: Inherit via back propagation
  Matrix Concatenation3 : Concatenate  NumInputs=3  Mode=Multidimensional array  ConcatenateDimension=2
  Switch{3..7} (5 alike) : Switch  Criteria=u2 ~= 0
  Signal : Outport
  "Merged " : Outport  Port=2
  wires:
  Switch6/1 -> "Merged "/1, Matrix Concatenation3/3
  Matrix Concatenation3/1 -> Signal/1
  Signal_avg/1 -> Switch7/1
  Merged_lane/1 -> Switch7/2
  Switch4/1 -> Matrix Concatenation3/2
  Switch3/1 -> Matrix Concatenation3/1
  Two_lanes/1 -> Switch4/2, Switch3/2
  Switch7/1 -> Switch6/3
  One_lane/1 -> Switch6/2
  Switch5/1 -> Switch6/1
  En_Left/1 -> Switch5/2
  Constant2/1 -> Switch7/3, Switch4/3, Switch3/3
  Signal_right/1 -> Switch5/3, Switch4/1
  Signal_left/1 -> Switch5/1, Switch3/1

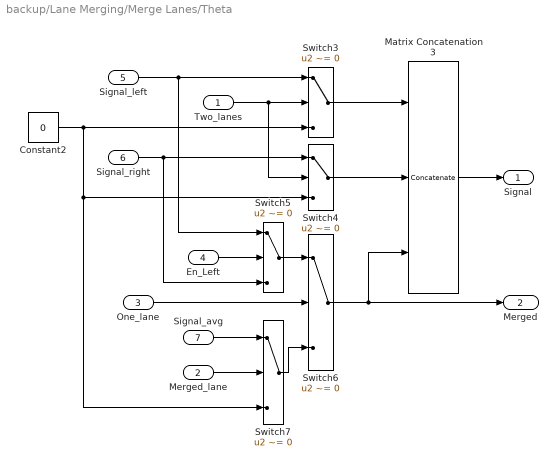
== system backup/Lane Merging/Merge Lanes/Theta ==
  Two_lanes : Inport
  Merged_lane : Inport  Port=2
  One_lane : Inport  Port=3
  En_Left : Inport  Port=4
  Signal_left : Inport  Port=5
  Signal_right : Inport  Port=6
  Signal_avg : Inport  Port=7
  Constant2 : Constant  Value=0  OutDataTypeStr=Inherit: Inherit via back propagation
  Matrix Concatenation3 : Concatenate  NumInputs=3  Mode=Multidimensional array  ConcatenateDimension=2
  Switch{3..7} (5 alike) : Switch  Criteria=u2 ~= 0
  Signal : Outport
  "Merged " : Outport  Port=2
  wires:
  Signal_left/1 -> Switch3/1, Switch5/1
  Signal_right/1 -> Switch4/1, Switch5/3
  Constant2/1 -> Switch3/3, Switch4/3, Switch7/3
  En_Left/1 -> Switch5/2
  Switch5/1 -> Switch6/1
  One_lane/1 -> Switch6/2
  Switch7/1 -> Switch6/3
  Two_lanes/1 -> Switch3/2, Switch4/2
  Switch3/1 -> Matrix Concatenation3/1
  Switch4/1 -> Matrix Concatenation3/2
  Merged_lane/1 -> Switch7/2
  Signal_avg/1 -> Switch7/1
  Matrix Concatenation3/1 -> Signal/1
  Switch6/1 -> Matrix Concatenation3/3, "Merged "/1

== matlab function backup/Lane Detection/Detection/Remove Undesired Chroma Pixels ==
  data: u input; y output
function y = ClearTopRight(u)
% Wipe out the top-right part of the image.

h = single(size(u, 1));
w = single(size(u, 2));
y = u;

step = h / w;
rs = single(0);
for c = 1: w
    for r = 1: round(rs)
        y(r, c) = 0;
    end
    rs = rs + step;
end

== matlab function backup/Lane Detection/Detection/Find Valid Pixels ==
  data: thr input; u input; y output
function y = FindValidPixels(thr, u)
%#codegen

[h, w] = size(u);
h_half = floor(h/2.0);
y = false(h, w);

for col = 1: w
    row = 1;
    acc = u(row, col);
    while acc < thr && row <= h_half
        y(row, col) = true;
        row = row + 1;
        acc = acc + u(row, col);
    end
    
    row = h;
    acc = u(row, col);
    while acc < thr && row > h_half
        y(row, col) = true;
        row = row - 1;
        acc = acc + u(row, col);
    end
end

== matlab function backup/Lane Detection/Right Side/Flip Right Region ==
  data: u input; y output
function y = FlipRight(u)
% Cut and flip the right part of the image

h = single(size(u, 1));
w = single(size(u, 2));
w_half = floor(w/2.0);
y = u(1:h, w:-1:w_half+1);

== matlab function backup/Lane Detection/Detection/Find First Strongest Edge ==
  data: u input; y output
function y = findMaxima(u)
% Find out the first local maxima

[h, w] = size(u);
half = floor(h/2.0);
y = single(zeros(h, w));

for c = 1: w
    r = 2;
    while r < half
        if u(r, c) > u(r-1, c) && u(r, c) > u(r+1, c)
            y(r, c) = u(r, c);
            break;
        end
        r = r + 1;
    end
    
    r = h-1;
    while r > half+1
        if u(r, c) > u(r-1, c) && u(r, c) > u(r+1, c)
            y(r, c) = u(r, c);
            break;
        end
        r = r - 1;
    end
end

== matlab function backup/Lane Detection/Left Side/Cut Left Region ==
  data: u input; y output
function y = CutLeft(u)
% Cut the left part of the image.

h = single(size(u, 1));
w = single(size(u, 2));
w_half = floor(w/2.0);
y = u(1:h, 1:w_half);

== matlab function backup/Lane Detection/Detection/Remove Undesired Edge Pixels ==
  data: u input; y output
function y = ClearTopRight(u)
% Wipe out the top-right part of the image.

h = single(size(u, 1));
w = single(size(u, 2));
y = u;

step = h / w;
rs = single(0);
for c = 1: w
    for r = 1: round(rs)
        y(r, c) = 0;
    end
    rs = rs + step;
end

== matlab function backup/Lane Detection/Left Side/Cut Left Edge ==
  data: u input; y output
function y = CutLeft(u)
% Cut the left part of the image.

h = single(size(u, 1));
w = single(size(u, 2));
w_half = floor(w/2.0);
y = u(1:h, 1:w_half);

== matlab function backup/Lane Detection/Right Side/Flip Right Edge ==
  data: u input; y output
function y = FlipRight(u)
% Cut and flip the right part of the image

h = single(size(u, 1));
w = single(size(u, 2));
w_half = floor(w/2.0);
y = u(1:h, w:-1:w_half+1);
